simulink model "Model_Segway"  (R2018a)
settings: Solver=FixedStepDiscrete  StartTime=0.0  StopTime=T_final  FixedStep=Ts  RelTol=1e-3
values from neighbouring files (symbols this model uses):
  dtheta_body_init = 0    [Run_Segway.m]
  theta_body_init = 0    [Run_Segway.m]
  theta_wheel_init = 0    [Run_Segway.m]
  torque = 0    [Run_Segway.m]
  Ts = 1/Fs    (= 0.005)    [Run_Segway.m]
settings Model: Creator=david  LastModifiedBy=david

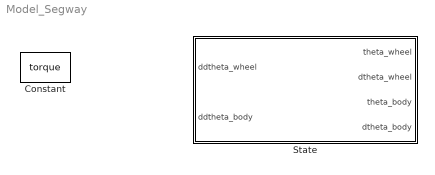
== system Model_Segway ==
  Constant : Constant  Value=torque
  State : Subsystem

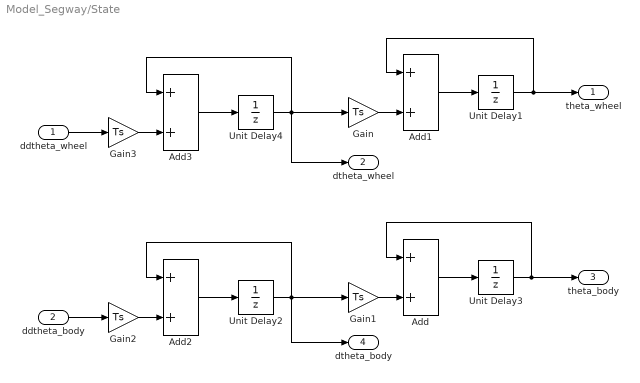
== system Model_Segway/State ==
  ddtheta_wheel : Inport
  ddtheta_body : Inport  Port=2
  Add{,1..3} (4 alike) : Sum
  Gain{,1..3} (4 alike) : Gain  Gain=Ts
  Unit Delay1 : UnitDelay  InitialCondition=theta_wheel_init  SampleTime=-1
  Unit Delay2 : UnitDelay  InitialCondition=dtheta_body_init  SampleTime=-1
  Unit Delay3 : UnitDelay  InitialCondition=theta_body_init  SampleTime=-1
  Unit Delay4 : UnitDelay  InitialCondition=dtheta_body_init  SampleTime=-1
  theta_wheel : Outport
  dtheta_wheel : Outport  Port=2
  theta_body : Outport  Port=3
  dtheta_body : Outport  Port=4
  wires:
  ddtheta_wheel/1 -> Gain3/1
  Unit Delay1/1 -> theta_wheel/1, Add1/1
  Unit Delay2/1 -> Gain1/1, dtheta_body/1, Add2/1
  Add/1 -> Unit Delay3/1
  Add1/1 -> Unit Delay1/1
  Unit Delay3/1 -> theta_body/1, Add/1
  Gain/1 -> Add1/2
  Gain1/1 -> Add/2
  ddtheta_body/1 -> Gain2/1
  Add2/1 -> Unit Delay2/1
  Gain2/1 -> Add2/2
  Unit Delay4/1 -> Gain/1, dtheta_wheel/1, Add3/1
  Add3/1 -> Unit Delay4/1
  Gain3/1 -> Add3/2
